simulink model "collect_data"  (R2012b)
settings: Solver=ode3  StartTime=0.0  StopTime=inf  FixedStep=0.001  RelTol=1e-3
settings Model: ExtModeTrigDuration=5000  Creator=paichihyun  LastModifiedBy=paichihyun
settings SolverCC: PositivePriorityOrder=on
settings RTWCC: SystemTargetFile=quarc_win64.tlc  TemplateMakefile=quarc_default_tmf  Description=QUARC Win64 Target  ProcessScript=quarc_win64_make_rtw_hook
settings STFCustomTargetCC: TargetPreCompLibLocation=C:\PROGRA~3\QUARC\lib\2012b\win64\release  CodeReplacementLibrary=ANSI_C  GeneratePreprocessorConditionals=Disable all  CombineOutputUpdateFcns=on  GRTInterface=off  SystemTargetFile=quarc_win64.tlc
settings GRTTargetCC: TargetPreCompLibLocation=C:\PROGRA~3\QUARC\lib\2012b\win64\release  ParMdlRefBuildCompliant=off  CompOptLevelCompliant=off  ConcurrentExecutionCompliant=off  MatFileLogging=off  ExtMode=on  ExtModeMexFile=quarc_comm

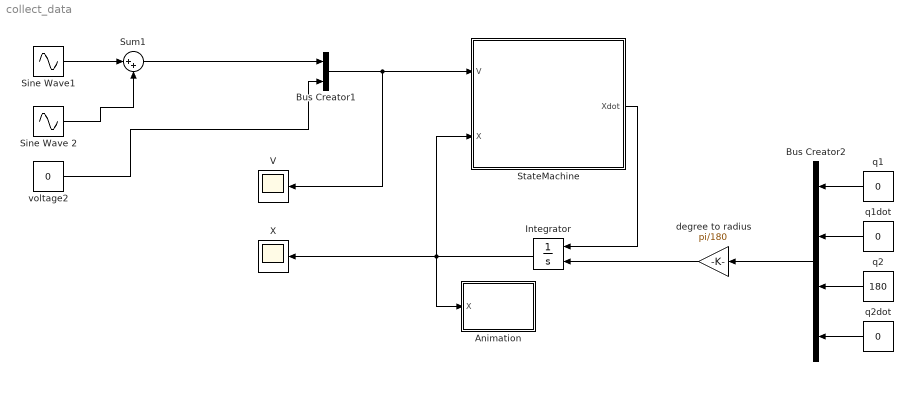
== system collect_data ==
  Animation : MATLAB Function  TreatAsAtomicUnit=on
  Bus Creator1 : BusCreator  Inputs=2
  Bus Creator2 : BusCreator
  Integrator : Integrator  InitialConditionSource=external
  Sine Wave 2 : Sin  Amplitude=7  Frequency=7  SampleTime=0
  Sine Wave1 : Sin  Amplitude=3  Frequency=3  SampleTime=0
  StateMachine : MATLAB Function  TreatAsAtomicUnit=on
  Sum1 : Sum  Inputs=|++
  V : Scope
      settings: SaveName=V_collect  MaxDataPoints=10800
  X : Scope
      settings: SaveName=X_collect  MaxDataPoints=10800
  degree to radius : Gain  Gain=pi/180
  q1 : Constant  Value=0
  q1dot : Constant  Value=0
  q2 : Constant  Value=180
  q2dot : Constant  Value=0
  voltage2 : Constant  Value=0
  wires:
  voltage2/1 -> Bus Creator1/2
  Bus Creator1/1 -> V/1, StateMachine/1(V)
  StateMachine/1(Xdot) -> Integrator/1
  Integrator/1 -> Animation/1(X), X/1, StateMachine/2(X)
  q1/1 -> Bus Creator2/1
  q1dot/1 -> Bus Creator2/2
  q2/1 -> Bus Creator2/3
  q2dot/1 -> Bus Creator2/4
  Bus Creator2/1 -> degree to radius/1
  degree to radius/1 -> Integrator/2
  Sum1/1 -> Bus Creator1/1
  Sine Wave1/1 -> Sum1/1
  Sine Wave 2/1 -> Sum1/2

== matlab function collect_data/Animation ==
  data: X input
function Animation(X)

theta1 = X(1);
theta2 = X(3);
% Sphere();
L1 = 6;
L2 = 2;
P0_Org=[0;0;0;1];
P1_Org=[0;0;-1;1];
P2_Org=[0;6;-1;1];
P3_Org=[0;6;0;1];
P4_Org=[0;8;0;1];
P5_Org=[0;12;0;1];

% theta1 = theta1 * pi / 180;
% theta2 = theta2 * pi / 180;

T01 = [cos(theta1),-sin(theta1),0,0;sin(theta1),cos(theta1),0,0;0,0,1,0;0,0,0,1];
P1 = T01 * P1_Org;
P2 = T01 * P2_Org;
P3 = T01 * P3_Org;
P4 = T01 * P4_Org;
T12 = [cos(theta2),-sin(theta2),0,0;0,0,-1,(L1+L2);sin(theta2),cos(theta2),0,0;0,0,0,1];
P5 = T01 * T12 * P5_Org;

plot3([P0_Org(1),P1(1),P2(1),P3(1),P4(1),P5(1)], [P0_Org(2),P1(2),P2(2),P3(2),P4(2),P5(2)], [P0_Org(3),P1(3),P2(3),P3(3),P4(3),P5(3)],'-o');
title('Robot Representation'); grid on;xlim([-10 10]);ylim([-10 10]);zlim([-10 10]);xlabel('x');ylabel('y');zlabel('z');
% drawnow
end

== matlab function collect_data/StateMachine ==
  data: V input; Xdot output; X input
function Xdot  =StateMachine(V, X)

% J1=0.0012;
% m2=0.127;
% l1_l2=0.2;
% l2=0.3;
% lc2=0.15;
% beta1=0.015;
% beta2=0.002;
% Ra=2.6;
% kt=0.00768;
% kv=0.00768;
% kr=70;
% 
% theta1=(J1+m2*l1_l2^2)*Ra/(kr*kt);
% theta2=(m2*l2^2/3)*Ra/(kr*kt);
% theta3=(m2*l1_l2*l2/2)*Ra/(kr*kt);

% theta4=(m2*lc2)*Ra/(kr*kt);
% theta5=beta1*Ra/(kr*kt) + kr*kv;
% theta6=beta2*Ra/(kr*kt);

q1=X(1);
q1dot=X(2);
q2=X(3);
q2dot=X(4);

theta1=0.030372023809524;
theta2=0.018426339285714;
theta3=0.018426339285714;
theta4=0.092131696428571;
theta5=0.610144642857143;
theta6=0.009672619047619;

m11=theta1+theta2*sin(q2)^2;
m12=theta3*cos(q2);
m21=theta3*cos(q2);
m22=theta2;
c11=2*theta2*sin(q2)*cos(q2)*q2dot;
c12=-theta3*sin(q2)*q2dot;
c21=-theta2*sin(q2)*cos(q2)*q1dot;
c22=0;
f1=theta5*q1dot;
f2=theta6*q2dot;                           
g=9.8;
g1=0;
g2=-theta4*g*sin(q2);

M=[m11,m12;m21,m22];
C=[c11,c12;c21,c22];
F=[f1;f2];
G=[g1;g2];
qdot=[q1dot;q2dot];

qdotdot=M\(V-C*qdot-F-G); 
Xdot=[q1dot,qdotdot(1),q2dot,qdotdot(2)];
Q=[q1;q2];
end
